simulink model "Cruise_model"  (R2020a)
settings: Solver=ode15s  StartTime=0.0  StopTime=30  MaxStep=0.1  RelTol=1e-3
values from neighbouring files (symbols this model uses):
  b = 50.0    [Ques_3_Parameters.sldd]
  m = 1000.0    [Ques_3_Parameters.sldd]
settings Model: DataDictionary=Ques_3_Parameters.sldd  Creator=DELL  LastModifiedBy=DELL

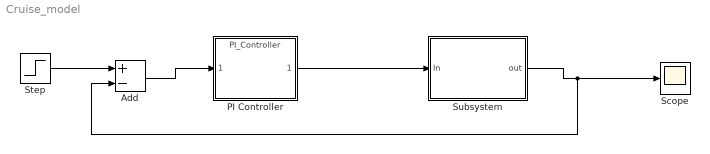
== system Cruise_model ==
  Add : Sum  Inputs=+-
  PI Controller : ModelReference  ModelNameDialog=PI_Controller  SimulationMode=Normal  ModelReferenceVersion=1.8
  Scope : Scope
  Step : Step  After=u  SampleTime=0
  Subsystem : Subsystem
  wires:
  Subsystem/1(out) -> Add/2, Scope/1
  PI Controller/1 -> Subsystem/1(In)
  Step/1 -> Add/1
  Add/1 -> PI Controller/1

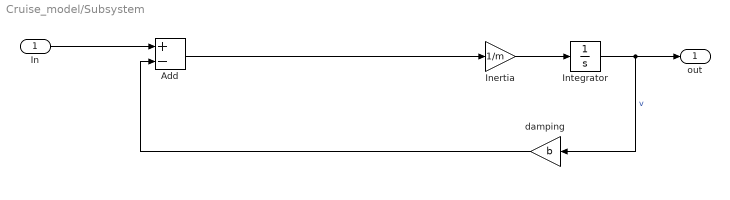
== system Cruise_model/Subsystem ==
  In : Inport
  Add : Sum  Inputs=+-
  Inertia : Gain  Gain=1/m
  Integrator : Integrator
  damping : Gain  Gain=b
  out : Outport
  wires:
  In/1 -> Add/1
  damping/1 -> Add/2
  Integrator/1 -> out/1, damping/1  "v"
  Inertia/1 -> Integrator/1
  Add/1 -> Inertia/1
